simulink library "hil_flowsensing_lib"  (R2019b)
settings: Solver=VariableStepAuto  StartTime=0.0  StopTime=10.0  RelTol=1e-3
libraries: simulink x2
settings Model: Creator=CentoPas  LastModifiedBy=CentoPas

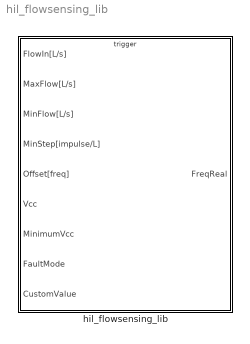
== system hil_flowsensing_lib ==
  hil_flowsensing_lib : Subsystem  TreatAsAtomicUnit=on  RTWFcnName=hil_flowsensing_lib  mask(Flow Meter){Parameter1={'FlowIn','single','0 to 10','L/s','Input water flow to be transduced';'MaxFlow','single','0 to max 32Bit','L/s','Maximum input flow due to hardware limits';'MinFlow','single','0 to MaxFlow','L/s','Minimum input flow to be detected by the sensor';'MinStep','single','0 to max 32Bit','impulse/L','Linear coefficient for flow - frequency transduction';'Offset','single','0 to max 32 Bit','Hz','Offset for linear dependency between flow and frequency for flow meter';'Vcc','single','0 to 5','V','Supply voltage';'MinimumVcc','single','0 to Vcc','V','Minimum supply voltage for flow meter functioning'}, Parameter2={'FaultMode','uint8','0 to 2','Adim','Simulate faults: 0 no fault, 1 no frequency, 2 custom value';'CustomValue','single','0 to maxfreq','Hz','Custom frequency value for fault managament'}, Parameter3={'FreqReal','single','0 to maxfreq','Hz','Output frequency of the flow meter, with fault management'}}
      mask help: The aim of this work is Model in Loop (MIL) testing of Flow Meter. It is here studied the case of a flow meter sensor, which is used mostly in washing machines for water pumping. The sensor transduces the water flow that comes in input as an output frequency, with the aim of regulating the amount of water which comes through. The transduction is expressed through a linear formula: frequency = Flow*Minstep + Offset. The correct functioning requires that the input flow is higher than a certain threshold, under which the sensor does not sense anything. Moreover, in the case the supply voltage is below the minimum requirement, the flow cannot be read. All threshold and linear formula parameters are tunable to fit to all possible future flow meters. Faults on output sensing are taken into account and simulated in the last block.
      settings: RTWFcnNameOpts=User specified
      mask Help: https://sdlcwiki.electrolux.com/display/ASTMBDHIL/Flow+Meter+@+EdmLib
      mask DialogControl Container5 Prompt: Inputs
      mask DialogControl Control2 Prompt: Fault Detection
      mask DialogControl Container6 Prompt: Outputs

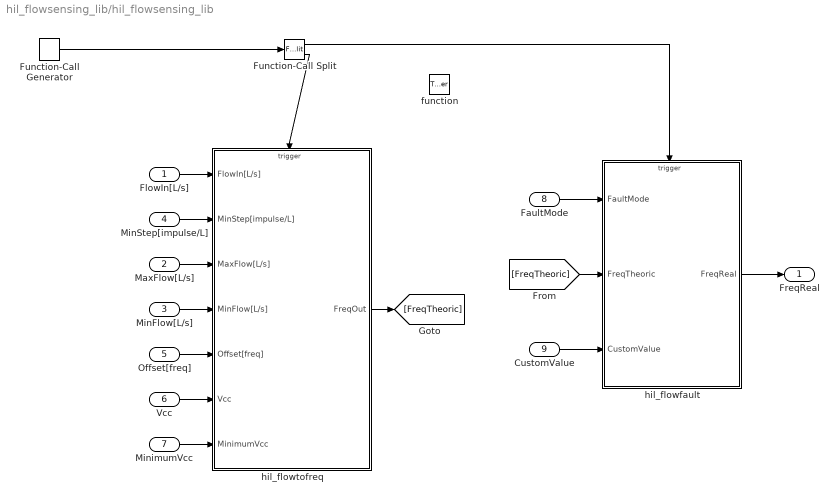
== system hil_flowsensing_lib/hil_flowsensing_lib ==
  FlowIn[L/s] : Inport
  MaxFlow[L/s] : Inport  Port=2
  MinFlow[L/s] : Inport  Port=3
  MinStep[impulse/L] : Inport  Port=4
  Offset[freq] : Inport  Port=5
  Vcc : Inport  Port=6
  MinimumVcc : Inport  Port=7
  FaultMode : Inport  Port=8
  CustomValue : Inport  Port=9
  function : TriggerPort  TriggerType=function-call  VariantControl=Variant
  Function-Call Generator : simulink/Ports & Subsystems/Function-Call Generator  sample_time=-1  numberOfIterations=1
  Function-Call Split : FunctionCallSplit  NumOutputPorts=2  OutputPortLayout=default
  hil_flowfault : Subsystem  TreatAsAtomicUnit=on
  hil_flowtofreq : Subsystem  TreatAsAtomicUnit=on
  FreqReal : Outport
  wires:
  Function-Call Generator/1 -> Function-Call Split/1
  Function-Call Split/2 -> hil_flowtofreq/Trigger
  Function-Call Split/1 -> hil_flowfault/Trigger
  hil_flowfault/1(FreqReal) -> FreqReal/1
  FlowIn[L/s]/1 -> hil_flowtofreq/1(FlowIn[L/s])
  FaultMode/1 -> hil_flowfault/1(FaultMode)
  hil_flowtofreq/1(FreqOut) -> [FreqTheoric]
  [FreqTheoric] -> hil_flowfault/2(FreqTheoric)
  CustomValue/1 -> hil_flowfault/3(CustomValue)
  MinStep[impulse/L]/1 -> hil_flowtofreq/2(MinStep[impulse/L])
  MaxFlow[L/s]/1 -> hil_flowtofreq/3(MaxFlow[L/s])
  MinFlow[L/s]/1 -> hil_flowtofreq/4(MinFlow[L/s])
  Vcc/1 -> hil_flowtofreq/6(Vcc)
  Offset[freq]/1 -> hil_flowtofreq/5(Offset[freq])
  MinimumVcc/1 -> hil_flowtofreq/7(MinimumVcc)

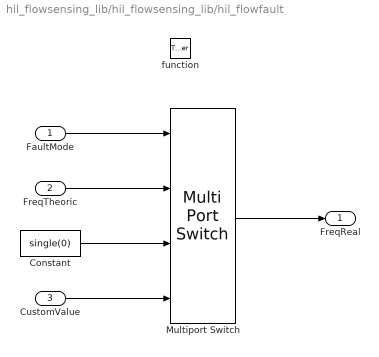
== system hil_flowsensing_lib/hil_flowsensing_lib/hil_flowfault ==
  FaultMode : Inport
  FreqTheoric : Inport  Port=2
  CustomValue : Inport  Port=3
  function : TriggerPort  TriggerType=function-call  VariantControl=Variant
  Constant : Constant  Value=single(0)
  Multiport Switch : MultiPortSwitch  DataPortOrder=Zero-based contiguous  DiagnosticForDefault=None  zeroidx=on
  FreqReal : Outport
  wires:
  Multiport Switch/1 -> FreqReal/1
  FaultMode/1 -> Multiport Switch/1
  FreqTheoric/1 -> Multiport Switch/2
  Constant/1 -> Multiport Switch/3
  CustomValue/1 -> Multiport Switch/4

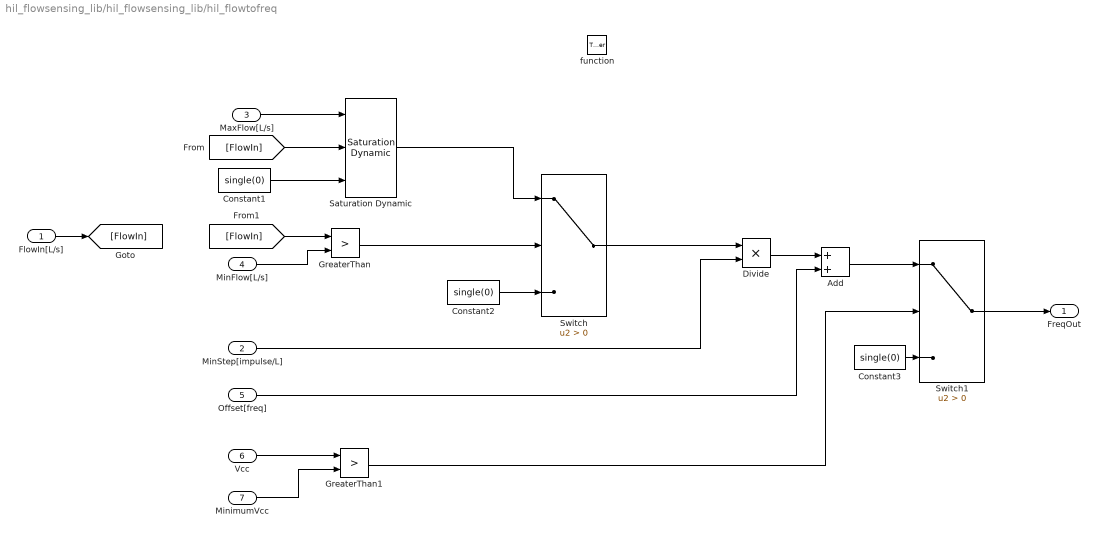
== system hil_flowsensing_lib/hil_flowsensing_lib/hil_flowtofreq ==
  FlowIn[L/s] : Inport
  MinStep[impulse/L] : Inport  Port=2
  MaxFlow[L/s] : Inport  Port=3
  MinFlow[L/s] : Inport  Port=4
  Offset[freq] : Inport  Port=5
  Vcc : Inport  Port=6
  MinimumVcc : Inport  Port=7
  function : TriggerPort  TriggerType=function-call  VariantControl=Variant
  Add : Sum
  Constant1 : Constant  Value=single(0)
  Constant2 : Constant  Value=single(0)
  Constant3 : Constant  Value=single(0)
  Divide : Product  Inputs=**
  GreaterThan : RelationalOperator  Operator=>  OutDataTypeStr=boolean  RndMeth=Simplest
  GreaterThan1 : RelationalOperator  Operator=>  OutDataTypeStr=boolean  RndMeth=Simplest
  Saturation Dynamic : simulink/Discontinuities/Saturation Dynamic  OutMin=[]  OutMax=[]  OutDataTypeStr=Inherit: Same as second input  OutDataType=fixdt(1, 16)  OutScaling=2^-10  DoSatur=off
  Switch : Switch  Criteria=u2 > Threshold
  Switch1 : Switch  Criteria=u2 > Threshold
  FreqOut : Outport
  wires:
  MinStep[impulse/L]/1 -> Divide/2
  MaxFlow[L/s]/1 -> Saturation Dynamic/1
  Constant1/1 -> Saturation Dynamic/3
  FlowIn[L/s]/1 -> [FlowIn]
  [FlowIn] -> Saturation Dynamic/2
  Switch/1 -> Divide/1
  Constant2/1 -> Switch/3
  [FlowIn] -> GreaterThan/1
  GreaterThan/1 -> Switch/2
  MinFlow[L/s]/1 -> GreaterThan/2
  Saturation Dynamic/1 -> Switch/1
  Divide/1 -> Add/1
  Offset[freq]/1 -> Add/2
  Switch1/1 -> FreqOut/1
  Add/1 -> Switch1/1
  Vcc/1 -> GreaterThan1/1
  MinimumVcc/1 -> GreaterThan1/2
  GreaterThan1/1 -> Switch1/2
  Constant3/1 -> Switch1/3
